simulink model "two_parallel_half_model_simscape"  (R2023b)
settings: Solver=ode1be  StartTime=0.0  StopTime=simlength  FixedStep=ts_sim  MaxStep=ts_sim
values from neighbouring files (symbols this model uses):
  fPWM_INV = 10e3    (= 10000)    [init_model.m]
  I_FS = Iout_ac_rms_nom * sqrt(2) * margin_factor    [init_model.m]
  ki_i_inv = 18    [init_model.m]
  ki_v_inv = 12.5    [init_model.m]
  kp_i_inv = 0.1    [init_model.m]
  kp_v_inv = 0.1    [init_model.m]
  LFu_ac = 125e-6*2    (= 0.00025)    [init_model.m]
  omega_grid = frequency_grid*2*pi    (= 314.159265359)    [init_model.m]
  RLFu_ac = 2e-3    (= 0.002)    [init_model.m]
  tc = ts_inv/200    (= 5e-07)    [init_model.m]
  ts_afe = ts_inv    (= 0.0001)    [init_model.m]
  ts_inv = tPWM_INV    (= 0.0001)    [init_model.m]
  ts_zvs = tPWM_ZVS*2    (= 0.0001)    [init_model.m]
  V_FS = Vout_dc_nom * margin_factor    (= 943)    [init_model.m]
  Vout_dc_nom = 820    [init_model.m]
undefined symbols (not defined in the file or in its folder): magnitude
libraries: fl_lib x43, nesl_utility x17
(part 2 of 2)

== system two_parallel_half_model_simscape/inverter_modB/single phase inverter/switch_1 ==
  Diode : fl_lib/Electrical/Electrical Elements/Diode  Vf=Vdon_diode V  Ron=Rdon_diode Ohm  Goff=1e-8 1/Ohm  i_specify=off  i_priority=None  i=0 A  i_nominal_specify=off  i_nominal_unit=A  i_nominal_value=1  v_specify=off  v_priority=None  v=0 V  v_nominal_specify=off  v_nominal_unit=V  v_nominal_value=1
  Switch : fl_lib/Electrical/Electrical Elements/Switch  R_closed=Ron Ohm  G_open=1e-8 1/Ohm  Threshold=7.5  i_specify=off  i_priority=None  i=0 A  i_nominal_specify=off  i_nominal_unit=A  i_nominal_value=1  v_specify=off  v_priority=None  v=0 V  v_nominal_specify=off  v_nominal_unit=V  v_nominal_value=1
  G : PMIOPort  Side=Left
  C : PMIOPort  Port=2  Side=Left
  E : PMIOPort  Port=3  Side=Right
  connections:
  Diode/LConn1 -- E/RConn1 -- Switch/LConn1
  Switch/RConn1 -- G/RConn1
  Diode/RConn1 -- C/RConn1 -- Switch/RConn2

== system two_parallel_half_model_simscape/inverter_modB/single phase inverter/switch_2 ==
  Diode : fl_lib/Electrical/Electrical Elements/Diode  Vf=Vdon_diode V  Ron=Rdon_diode Ohm  Goff=1e-8 1/Ohm  i_specify=off  i_priority=None  i=0 A  i_nominal_specify=off  i_nominal_unit=A  i_nominal_value=1  v_specify=off  v_priority=None  v=0 V  v_nominal_specify=off  v_nominal_unit=V  v_nominal_value=1
  Switch : fl_lib/Electrical/Electrical Elements/Switch  R_closed=Ron Ohm  G_open=1e-8 1/Ohm  Threshold=7.5  i_specify=off  i_priority=None  i=0 A  i_nominal_specify=off  i_nominal_unit=A  i_nominal_value=1  v_specify=off  v_priority=None  v=0 V  v_nominal_specify=off  v_nominal_unit=V  v_nominal_value=1
  G : PMIOPort  Side=Left
  C : PMIOPort  Port=2  Side=Left
  E : PMIOPort  Port=3  Side=Right
  connections:
  Switch/RConn2 -- C/RConn1 -- Diode/RConn1
  Switch/RConn1 -- G/RConn1
  Switch/LConn1 -- E/RConn1 -- Diode/LConn1

== system two_parallel_half_model_simscape/inverter_modB/single phase inverter/switch_3 ==
  Diode : fl_lib/Electrical/Electrical Elements/Diode  Vf=Vdon_diode V  Ron=Rdon_diode Ohm  Goff=1e-8 1/Ohm  i_specify=off  i_priority=None  i=0 A  i_nominal_specify=off  i_nominal_unit=A  i_nominal_value=1  v_specify=off  v_priority=None  v=0 V  v_nominal_specify=off  v_nominal_unit=V  v_nominal_value=1
  Switch : fl_lib/Electrical/Electrical Elements/Switch  R_closed=Ron Ohm  G_open=1e-8 1/Ohm  Threshold=7.5  i_specify=off  i_priority=None  i=0 A  i_nominal_specify=off  i_nominal_unit=A  i_nominal_value=1  v_specify=off  v_priority=None  v=0 V  v_nominal_specify=off  v_nominal_unit=V  v_nominal_value=1
  G : PMIOPort  Side=Left
  C : PMIOPort  Port=2  Side=Left
  E : PMIOPort  Port=3  Side=Right
  connections:
  Diode/LConn1 -- E/RConn1 -- Switch/LConn1
  Switch/RConn1 -- G/RConn1
  Diode/RConn1 -- C/RConn1 -- Switch/RConn2

== system two_parallel_half_model_simscape/inverter_modB/single phase inverter/switch_4 ==
  Diode : fl_lib/Electrical/Electrical Elements/Diode  Vf=Vdon_diode V  Ron=Rdon_diode Ohm  Goff=1e-8 1/Ohm  i_specify=off  i_priority=None  i=0 A  i_nominal_specify=off  i_nominal_unit=A  i_nominal_value=1  v_specify=off  v_priority=None  v=0 V  v_nominal_specify=off  v_nominal_unit=V  v_nominal_value=1
  Switch : fl_lib/Electrical/Electrical Elements/Switch  R_closed=Ron Ohm  G_open=1e-8 1/Ohm  Threshold=7.5  i_specify=off  i_priority=None  i=0 A  i_nominal_specify=off  i_nominal_unit=A  i_nominal_value=1  v_specify=off  v_priority=None  v=0 V  v_nominal_specify=off  v_nominal_unit=V  v_nominal_value=1
  G : PMIOPort  Side=Left
  C : PMIOPort  Port=2  Side=Left
  E : PMIOPort  Port=3  Side=Right
  connections:
  Switch/RConn2 -- C/RConn1 -- Diode/RConn1
  Switch/RConn1 -- G/RConn1
  Switch/LConn1 -- E/RConn1 -- Diode/LConn1

== system two_parallel_half_model_simscape/inverter_modB/single phase inverter control/acquisition_and_scaling_current ==
  in : Inport
  1/Ti5 : Gain  Gain=1/I_FS  SaturateOnIntegerOverflow=on  OutDataTypeStr=Inherit: Same as input  ParamDataTypeStr=Inherit: Same as input
  Unit Delay4 : UnitDelay  SampleTime=ts_inv  HasFrameUpgradeWarning=on
  Zero-Order Hold1 : ZeroOrderHold  SampleTime=ts_inv
  out : Outport
  wires:
  Unit Delay4/1 -> out/1
  Zero-Order Hold1/1 -> 1/Ti5/1
  1/Ti5/1 -> Unit Delay4/1
  in/1 -> Zero-Order Hold1/1

== system two_parallel_half_model_simscape/inverter_modB/single phase inverter control/alphabeta2dq ==
  note: va=V cos(wt)
      | vb=V cos(wt-2pi/3)
      | vc=V cos(wt+2pi/3)
  alpha : Inport
  beta : Inport  Port=2
  wt : Inport  Port=3
  Product{,1..3} (4 alike) : Product  RndMeth=Zero
  Sum : Sum
  Sum1 : Sum  Inputs=-+
  To Workspace1 : ToWorkspace  VariableName=id_pu_modB_sim  SampleTime=ts_inv
      settings: MaxDataPoints=Ns_inv
  To Workspace2 : ToWorkspace  VariableName=iq_pu_modB_sim  SampleTime=ts_inv
      settings: MaxDataPoints=Ns_inv
  Trigonometric Function : Trigonometry  Operator=cos
  Trigonometric Function1 : Trigonometry
  "d " : Outport  VectorParamsAs1DForOutWhenUnconnected=off
  "q " : Outport  Port=2  VectorParamsAs1DForOutWhenUnconnected=off
  wires:
  Sum1/1 -> "q "/1, To Workspace2/1
  [cos] -> Product3/1
  Product3/1 -> Sum1/2
  Product2/1 -> Sum1/1
  [sin] -> Product2/1
  Sum/1 -> "d "/1, To Workspace1/1
  beta/1 -> Product3/2, Product1/2
  [sin] -> Product1/1
  Product1/1 -> Sum/2
  Product/1 -> Sum/1
  alpha/1 -> Product2/2, Product/2
  [cos] -> Product/1
  Trigonometric Function1/1 -> [sin]
  Trigonometric Function/1 -> [cos]
  wt/1 -> Trigonometric Function/1, Trigonometric Function1/1

== system two_parallel_half_model_simscape/inverter_modB/single phase inverter control/dq2alphabeta ==
  d : Inport
  q : Inport  Port=2
  wt : Inport  Port=3
  Product{,1..3} (4 alike) : Product  RndMeth=Zero
  Sum : Sum  Inputs=+-
  Sum1 : Sum
  Trigonometric Function : Trigonometry  Operator=cos
  Trigonometric Function1 : Trigonometry
  alpha : Outport  VectorParamsAs1DForOutWhenUnconnected=off
  wires:
  wt/1 -> Trigonometric Function1/1, Trigonometric Function/1
  Trigonometric Function/1 -> [cos]
  Trigonometric Function1/1 -> [sin]
  [cos] -> Product/1
  d/1 -> Product/2, Product2/2
  Product/1 -> Sum/1
  Product1/1 -> Sum/2
  [sin] -> Product1/1
  q/1 -> Product1/2, Product3/2
  Sum/1 -> alpha/1
  [sin] -> Product2/1
  Product2/1 -> Sum1/1
  Product3/1 -> Sum1/2
  [cos] -> Product3/1

== system two_parallel_half_model_simscape/inverter_modB/single phase inverter control/pi_d ==
  id_tilde : Inport
  1/Ti : Gain  Gain=kp_i_inv  SaturateOnIntegerOverflow=on  OutDataTypeStr=Inherit: Same as input  ParamDataTypeStr=Inherit: Same as input
  Sum1 : Sum  Inputs=+++  SaturateOnIntegerOverflow=on
  Sum3 : Sum  Inputs=-+  SaturateOnIntegerOverflow=on
  To Workspace3 : ToWorkspace  VariableName=id_ctrl_out_modB_sim  SampleTime=ts_inv
      settings: MaxDataPoints=Ns_inv
  Unit Delay4 : UnitDelay  SampleTime=ts_inv  HasFrameUpgradeWarning=on
  kp2 : Gain  Gain=ki_i_inv*ts_inv  SaturateOnIntegerOverflow=on  OutDataTypeStr=Inherit: Same as input  ParamDataTypeStr=Inherit: Same as input
  ud_out_lim : Saturate  UpperLimit=1  LowerLimit=-1
  "ud_out_lim " : Saturate  UpperLimit=1  LowerLimit=-1
  Vd_out : Outport  VectorParamsAs1DForOutWhenUnconnected=off
  wires:
  "ud_out_lim "/1 -> Vd_out/1, To Workspace3/1
  ud_out_lim/1 -> "ud_out_lim "/1, Sum3/2
  Sum3/1 -> Unit Delay4/1
  Unit Delay4/1 -> Sum1/3
  1/Ti/1 -> Sum3/1, Sum1/1
  kp2/1 -> Sum1/2
  Sum1/1 -> ud_out_lim/1
  id_tilde/1 -> 1/Ti/1, kp2/1

== system two_parallel_half_model_simscape/inverter_modB/single phase inverter control/pi_q ==
  iq_tilde : Inport
  1/Ti : Gain  Gain=kp_i_inv  SaturateOnIntegerOverflow=on  OutDataTypeStr=Inherit: Same as input  ParamDataTypeStr=Inherit: Same as input
  Sum1 : Sum  Inputs=+++  SaturateOnIntegerOverflow=on
  Sum3 : Sum  Inputs=-+  SaturateOnIntegerOverflow=on
  To Workspace3 : ToWorkspace  VariableName=iq_ctrl_out_modB_sim  SampleTime=ts_inv
      settings: MaxDataPoints=Ns_inv
  Unit Delay4 : UnitDelay  SampleTime=ts_inv  HasFrameUpgradeWarning=on
  kp2 : Gain  Gain=ki_i_inv*ts_inv  SaturateOnIntegerOverflow=on  OutDataTypeStr=Inherit: Same as input  ParamDataTypeStr=Inherit: Same as input
  ud_out_lim : Saturate  UpperLimit=1  LowerLimit=-1
  "uq_out_lim " : Saturate  UpperLimit=1  LowerLimit=-1
  Vd_out : Outport  VectorParamsAs1DForOutWhenUnconnected=off
  wires:
  Sum1/1 -> ud_out_lim/1
  kp2/1 -> Sum1/2
  1/Ti/1 -> Sum1/1, Sum3/1
  Unit Delay4/1 -> Sum1/3
  Sum3/1 -> Unit Delay4/1
  ud_out_lim/1 -> Sum3/2, "uq_out_lim "/1
  "uq_out_lim "/1 -> To Workspace3/1, Vd_out/1
  iq_tilde/1 -> kp2/1, 1/Ti/1

== system two_parallel_half_model_simscape/inverter_modB/single phase inverter control/pwm ==
  vout : Inport
  Constant : Constant  Value=pi/12
  Constant1 : Constant
  Constant2 : Constant
  Constant3 : Constant
  Gain1 : Gain  Gain=1/2
  Gain2 : Gain
  Gain3 : Gain  Gain=1/2
  Gain4 : Gain  Gain=-1
  PWM generator 1 : Subsystem  mask{f=fPWM_INV, m_up=1, m_low=0, dead_time=0, pos_cmd_gate=15, neg_cmd_gate=-10, polarity=-1}
      mask prompts: f "Frequency (Hz)"; m_up "Max Input Modulation Value"; m_low "Min Input Modulation Value"; dead_time "Dead Time (s)"; pos_cmd_gate "Positive Gate Voltage (V)"; neg_cmd_gate "Negative Gate Voltage (V)"; polarity "Polarity (pu)"
  PWM generator 2 : Subsystem  mask{f=fPWM_INV, m_up=1, m_low=0, dead_time=0, pos_cmd_gate=15, neg_cmd_gate=-10, polarity=-1}
      mask prompts: f "Frequency (Hz)"; m_up "Max Input Modulation Value"; m_low "Min Input Modulation Value"; dead_time "Dead Time (s)"; pos_cmd_gate "Positive Gate Voltage (V)"; neg_cmd_gate "Negative Gate Voltage (V)"; polarity "Polarity (pu)"
  Sum : Sum  Inputs=|++
  Sum1 : Sum  Inputs=|++
  m1_top : Outport
  m1_bottom : Outport  Port=2
  m2_top : Outport  Port=3
  m2_bottom : Outport  Port=4
  wires:
  PWM generator 1/1(m1) -> m1_top/1  "gate_cmd_Q1"
  PWM generator 1/2(m2) -> m1_bottom/1  "gate_cmd_Q2"
  PWM generator 2/2(m2) -> m2_bottom/1  "gate_cmd_Q2"
  PWM generator 2/1(m1) -> m2_top/1  "gate_cmd_Q1"
  Constant/1 -> PWM generator 2/2(phase), PWM generator 1/2(phase)
  Constant1/1 -> PWM generator 2/3(polarity_input), PWM generator 1/3(polarity_input)
  Gain2/1 -> Sum/1
  Sum/1 -> Gain1/1
  Constant2/1 -> Sum/2
  Gain1/1 -> PWM generator 1/1(m_index)
  Constant3/1 -> Sum1/2
  Sum1/1 -> Gain3/1
  Gain4/1 -> Sum1/1
  Gain3/1 -> PWM generator 2/1(m_index)
  vout/1 -> Gain4/1, Gain2/1

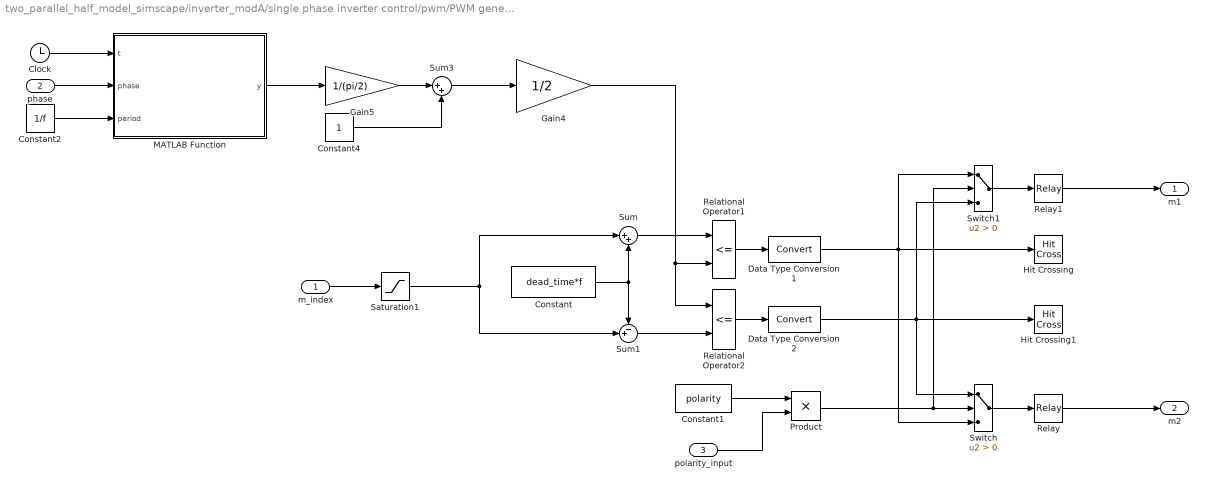
== system two_parallel_half_model_simscape/inverter_modA/single phase inverter control/pwm/PWM generator 1 ==
  m_index : Inport
  phase : Inport  Port=2
  polarity_input : Inport  Port=3
  Clock : Clock
  Constant : Constant  Value=dead_time*f
  Constant1 : Constant  Value=polarity
  Constant2 : Constant  Value=1/f
  Constant4 : Constant
  Data Type Conversion1 : DataTypeConversion
  Data Type Conversion2 : DataTypeConversion
  Gain4 : Gain  Gain=1/2
  Gain5 : Gain  Gain=1/(pi/2)
  Hit Crossing : HitCross  ShowOutputPort=off
  Hit Crossing1 : HitCross  ShowOutputPort=off
  MATLAB Function : MATLAB Function  TreatAsAtomicUnit=on
  Product : Product
  Relational Operator1 : RelationalOperator  Operator=<=  InputSameDT=off
  Relational Operator2 : RelationalOperator  Operator=<=  InputSameDT=off
  Relay : Relay  OnOutputValue=pos_cmd_gate  OffOutputValue=neg_cmd_gate
  Relay1 : Relay  OnOutputValue=pos_cmd_gate  OffOutputValue=neg_cmd_gate
  Saturation1 : Saturate  UpperLimit=m_up  LowerLimit=m_low
  Sum : Sum  Inputs=|++  SaturateOnIntegerOverflow=on
  Sum1 : Sum  Inputs=-+|  SaturateOnIntegerOverflow=on
  Sum3 : Sum  Inputs=|++
  Switch : Switch  Criteria=u2 > Threshold  SaturateOnIntegerOverflow=off  InputSameDT=off
  Switch1 : Switch  Criteria=u2 > Threshold  SaturateOnIntegerOverflow=off  InputSameDT=off
  m1 : Outport
  m2 : Outport  Port=2
  wires:
  Relational Operator1/1 -> Data Type Conversion1/1
  m_index/1 -> Saturation1/1
  Relational Operator2/1 -> Data Type Conversion2/1
  Data Type Conversion2/1 -> Switch/1, Switch1/3, Hit Crossing1/1
  Constant/1 -> Sum/2, Sum1/1
  Saturation1/1 -> Sum/1, Sum1/2
  Sum/1 -> Relational Operator1/1
  Sum1/1 -> Relational Operator2/2
  Gain4/1 -> Relational Operator2/1, Relational Operator1/2
  Data Type Conversion1/1 -> Hit Crossing/1, Switch/3, Switch1/1
  Switch/1 -> Relay/1
  Clock/1 -> MATLAB Function/1(t)
  Constant2/1 -> MATLAB Function/3(period)
  phase/1 -> MATLAB Function/2(phase)
  MATLAB Function/1(y) -> Gain5/1
  Gain5/1 -> Sum3/1
  Sum3/1 -> Gain4/1
  Constant4/1 -> Sum3/2
  Relay/1 -> m2/1
  Product/1 -> Switch1/2, Switch/2
  Switch1/1 -> Relay1/1
  Relay1/1 -> m1/1
  Constant1/1 -> Product/1
  polarity_input/1 -> Product/2

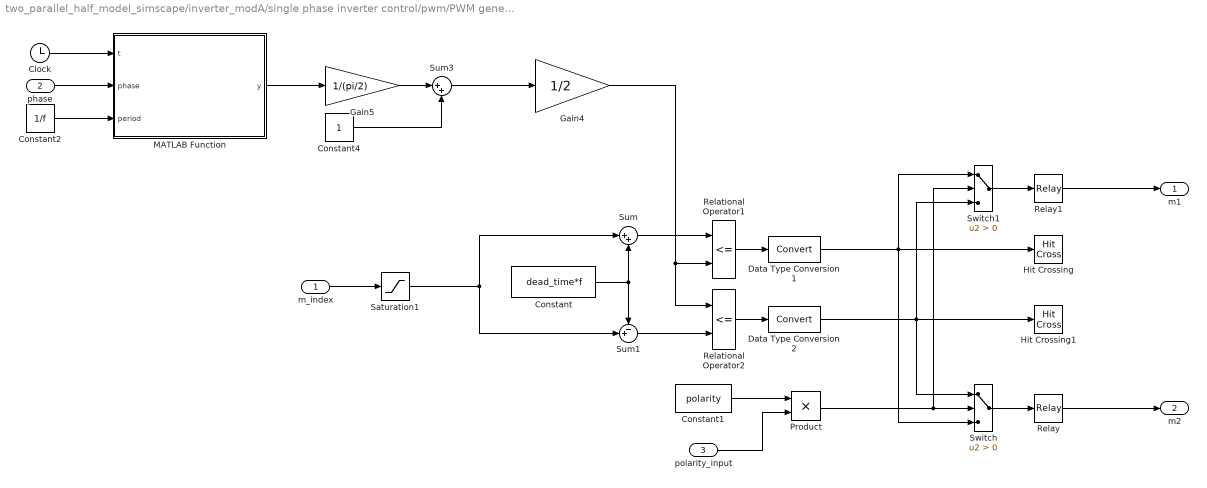
== system two_parallel_half_model_simscape/inverter_modA/single phase inverter control/pwm/PWM generator 2 ==
  m_index : Inport
  phase : Inport  Port=2
  polarity_input : Inport  Port=3
  Clock : Clock
  Constant : Constant  Value=dead_time*f
  Constant1 : Constant  Value=polarity
  Constant2 : Constant  Value=1/f
  Constant4 : Constant
  Data Type Conversion1 : DataTypeConversion
  Data Type Conversion2 : DataTypeConversion
  Gain4 : Gain  Gain=1/2
  Gain5 : Gain  Gain=1/(pi/2)
  Hit Crossing : HitCross  ShowOutputPort=off
  Hit Crossing1 : HitCross  ShowOutputPort=off
  MATLAB Function : MATLAB Function  TreatAsAtomicUnit=on
  Product : Product
  Relational Operator1 : RelationalOperator  Operator=<=  InputSameDT=off
  Relational Operator2 : RelationalOperator  Operator=<=  InputSameDT=off
  Relay : Relay  OnOutputValue=pos_cmd_gate  OffOutputValue=neg_cmd_gate
  Relay1 : Relay  OnOutputValue=pos_cmd_gate  OffOutputValue=neg_cmd_gate
  Saturation1 : Saturate  UpperLimit=m_up  LowerLimit=m_low
  Sum : Sum  Inputs=|++  SaturateOnIntegerOverflow=on
  Sum1 : Sum  Inputs=-+|  SaturateOnIntegerOverflow=on
  Sum3 : Sum  Inputs=|++
  Switch : Switch  Criteria=u2 > Threshold  SaturateOnIntegerOverflow=off  InputSameDT=off
  Switch1 : Switch  Criteria=u2 > Threshold  SaturateOnIntegerOverflow=off  InputSameDT=off
  m1 : Outport
  m2 : Outport  Port=2
  wires:
  polarity_input/1 -> Product/2
  Constant1/1 -> Product/1
  Relay1/1 -> m1/1
  Switch1/1 -> Relay1/1
  Product/1 -> Switch/2, Switch1/2
  Relay/1 -> m2/1
  Constant4/1 -> Sum3/2
  Sum3/1 -> Gain4/1
  Gain5/1 -> Sum3/1
  MATLAB Function/1(y) -> Gain5/1
  phase/1 -> MATLAB Function/2(phase)
  Constant2/1 -> MATLAB Function/3(period)
  Clock/1 -> MATLAB Function/1(t)
  Switch/1 -> Relay/1
  Data Type Conversion1/1 -> Switch1/1, Switch/3, Hit Crossing/1
  Gain4/1 -> Relational Operator1/2, Relational Operator2/1
  Sum1/1 -> Relational Operator2/2
  Sum/1 -> Relational Operator1/1
  Saturation1/1 -> Sum1/2, Sum/1
  Constant/1 -> Sum1/1, Sum/2
  Data Type Conversion2/1 -> Hit Crossing1/1, Switch1/3, Switch/1
  Relational Operator2/1 -> Data Type Conversion2/1
  m_index/1 -> Saturation1/1
  Relational Operator1/1 -> Data Type Conversion1/1

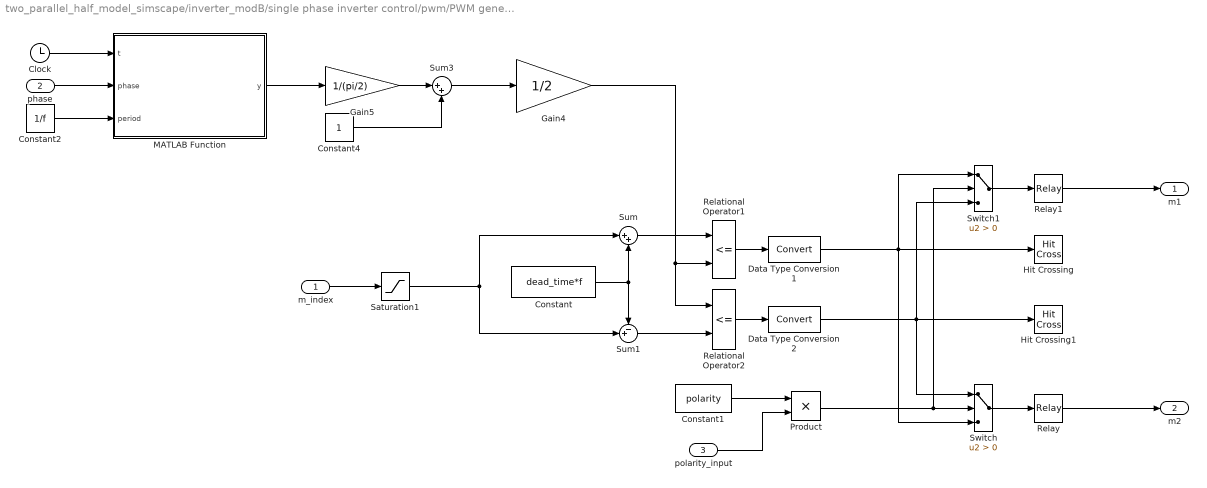
== system two_parallel_half_model_simscape/inverter_modB/single phase inverter control/pwm/PWM generator 1 ==
  m_index : Inport
  phase : Inport  Port=2
  polarity_input : Inport  Port=3
  Clock : Clock
  Constant : Constant  Value=dead_time*f
  Constant1 : Constant  Value=polarity
  Constant2 : Constant  Value=1/f
  Constant4 : Constant
  Data Type Conversion1 : DataTypeConversion
  Data Type Conversion2 : DataTypeConversion
  Gain4 : Gain  Gain=1/2
  Gain5 : Gain  Gain=1/(pi/2)
  Hit Crossing : HitCross  ShowOutputPort=off
  Hit Crossing1 : HitCross  ShowOutputPort=off
  MATLAB Function : MATLAB Function  TreatAsAtomicUnit=on
  Product : Product
  Relational Operator1 : RelationalOperator  Operator=<=  InputSameDT=off
  Relational Operator2 : RelationalOperator  Operator=<=  InputSameDT=off
  Relay : Relay  OnOutputValue=pos_cmd_gate  OffOutputValue=neg_cmd_gate
  Relay1 : Relay  OnOutputValue=pos_cmd_gate  OffOutputValue=neg_cmd_gate
  Saturation1 : Saturate  UpperLimit=m_up  LowerLimit=m_low
  Sum : Sum  Inputs=|++  SaturateOnIntegerOverflow=on
  Sum1 : Sum  Inputs=-+|  SaturateOnIntegerOverflow=on
  Sum3 : Sum  Inputs=|++
  Switch : Switch  Criteria=u2 > Threshold  SaturateOnIntegerOverflow=off  InputSameDT=off
  Switch1 : Switch  Criteria=u2 > Threshold  SaturateOnIntegerOverflow=off  InputSameDT=off
  m1 : Outport
  m2 : Outport  Port=2
  wires:
  Relational Operator1/1 -> Data Type Conversion1/1
  m_index/1 -> Saturation1/1
  Relational Operator2/1 -> Data Type Conversion2/1
  Data Type Conversion2/1 -> Switch/1, Switch1/3, Hit Crossing1/1
  Constant/1 -> Sum/2, Sum1/1
  Saturation1/1 -> Sum/1, Sum1/2
  Sum/1 -> Relational Operator1/1
  Sum1/1 -> Relational Operator2/2
  Gain4/1 -> Relational Operator2/1, Relational Operator1/2
  Data Type Conversion1/1 -> Hit Crossing/1, Switch/3, Switch1/1
  Switch/1 -> Relay/1
  Clock/1 -> MATLAB Function/1(t)
  Constant2/1 -> MATLAB Function/3(period)
  phase/1 -> MATLAB Function/2(phase)
  MATLAB Function/1(y) -> Gain5/1
  Gain5/1 -> Sum3/1
  Sum3/1 -> Gain4/1
  Constant4/1 -> Sum3/2
  Relay/1 -> m2/1
  Product/1 -> Switch1/2, Switch/2
  Switch1/1 -> Relay1/1
  Relay1/1 -> m1/1
  Constant1/1 -> Product/1
  polarity_input/1 -> Product/2

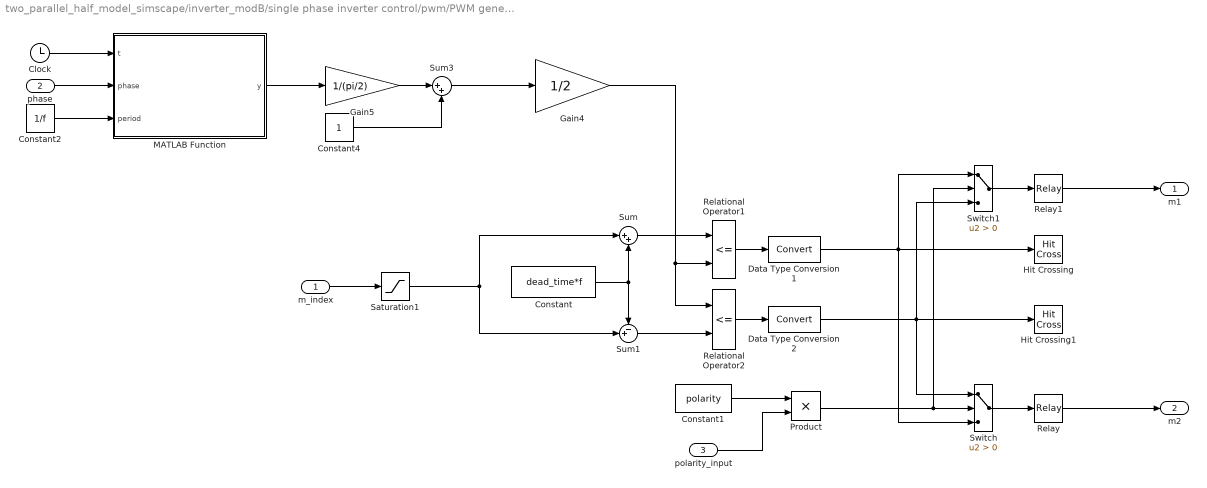
== system two_parallel_half_model_simscape/inverter_modB/single phase inverter control/pwm/PWM generator 2 ==
  m_index : Inport
  phase : Inport  Port=2
  polarity_input : Inport  Port=3
  Clock : Clock
  Constant : Constant  Value=dead_time*f
  Constant1 : Constant  Value=polarity
  Constant2 : Constant  Value=1/f
  Constant4 : Constant
  Data Type Conversion1 : DataTypeConversion
  Data Type Conversion2 : DataTypeConversion
  Gain4 : Gain  Gain=1/2
  Gain5 : Gain  Gain=1/(pi/2)
  Hit Crossing : HitCross  ShowOutputPort=off
  Hit Crossing1 : HitCross  ShowOutputPort=off
  MATLAB Function : MATLAB Function  TreatAsAtomicUnit=on
  Product : Product
  Relational Operator1 : RelationalOperator  Operator=<=  InputSameDT=off
  Relational Operator2 : RelationalOperator  Operator=<=  InputSameDT=off
  Relay : Relay  OnOutputValue=pos_cmd_gate  OffOutputValue=neg_cmd_gate
  Relay1 : Relay  OnOutputValue=pos_cmd_gate  OffOutputValue=neg_cmd_gate
  Saturation1 : Saturate  UpperLimit=m_up  LowerLimit=m_low
  Sum : Sum  Inputs=|++  SaturateOnIntegerOverflow=on
  Sum1 : Sum  Inputs=-+|  SaturateOnIntegerOverflow=on
  Sum3 : Sum  Inputs=|++
  Switch : Switch  Criteria=u2 > Threshold  SaturateOnIntegerOverflow=off  InputSameDT=off
  Switch1 : Switch  Criteria=u2 > Threshold  SaturateOnIntegerOverflow=off  InputSameDT=off
  m1 : Outport
  m2 : Outport  Port=2
  wires:
  polarity_input/1 -> Product/2
  Constant1/1 -> Product/1
  Relay1/1 -> m1/1
  Switch1/1 -> Relay1/1
  Product/1 -> Switch/2, Switch1/2
  Relay/1 -> m2/1
  Constant4/1 -> Sum3/2
  Sum3/1 -> Gain4/1
  Gain5/1 -> Sum3/1
  MATLAB Function/1(y) -> Gain5/1
  phase/1 -> MATLAB Function/2(phase)
  Constant2/1 -> MATLAB Function/3(period)
  Clock/1 -> MATLAB Function/1(t)
  Switch/1 -> Relay/1
  Data Type Conversion1/1 -> Switch1/1, Switch/3, Hit Crossing/1
  Gain4/1 -> Relational Operator1/2, Relational Operator2/1
  Sum1/1 -> Relational Operator2/2
  Sum/1 -> Relational Operator1/1
  Saturation1/1 -> Sum1/2, Sum/1
  Constant/1 -> Sum1/1, Sum/2
  Data Type Conversion2/1 -> Hit Crossing1/1, Switch1/3, Switch/1
  Relational Operator2/1 -> Data Type Conversion2/1
  m_index/1 -> Saturation1/1
  Relational Operator1/1 -> Data Type Conversion1/1

== matlab function two_parallel_half_model_simscape/inverter_modA/single phase inverter control/pwm/PWM generator 2/MATLAB Function ==
  data: t input; y output; phase input; period input
function y = trgo(t,phase,period)
x = sin(2*pi/period*t - phase - pi/2);
y = asin(x);

== matlab function two_parallel_half_model_simscape/inverter_modB/single phase inverter control/flt_dq_d_i1 ==
  data: input input; y output
function y  = flt_dq_d(input)

FLTD2Q_B1 = 0.000966531084866133;
FLTD2Q_B2 = 0.000946498544476605;
FLTD2Q_A1 = -1.93814485260962;
FLTD2Q_A2 = 0.939101367424292;

    persistent x1 x2 y1 y2

    if isempty(x1)
        x1=0;
        x2=0;
        y1=0;
        y2=0;
    end


    o = x1 * FLTD2Q_B1 + x2 * FLTD2Q_B2 - y1 * FLTD2Q_A1 - y2 * FLTD2Q_A2;
    x2 = x1;
    x1 = input;
    y2 = y1;
    y1 = o;
	y = o;
end

== matlab function two_parallel_half_model_simscape/inverter_modA/phase_gen/bounder1 ==
  data: u input; y output
function y = bounder(u)
    
    y = -pi + mod(u+3*pi,2*pi);
end

== matlab function two_parallel_half_model_simscape/inverter_modA/single phase inverter control/flt_dq_d_i ==
  data: input input; y output
function y  = flt_dq_d(input)

FLTD2Q_B1 = 0.000966531084866133;
FLTD2Q_B2 = 0.000946498544476605;
FLTD2Q_A1 = -1.93814485260962;
FLTD2Q_A2 = 0.939101367424292;

    persistent x1 x2 y1 y2

    if isempty(x1)
        x1=0;
        x2=0;
        y1=0;
        y2=0;
    end


    o = x1 * FLTD2Q_B1 + x2 * FLTD2Q_B2 - y1 * FLTD2Q_A1 - y2 * FLTD2Q_A2;
    x2 = x1;
    x1 = input;
    y2 = y1;
    y1 = o;
	y = o;
end

== matlab function two_parallel_half_model_simscape/inverter_modA/single phase inverter control/flt_dq_d_u ==
  data: input input; y output
function y  = flt_dq_d(input)

FLTD2Q_B1 = 0.000966531084866133;
FLTD2Q_B2 = 0.000946498544476605;
FLTD2Q_A1 = -1.93814485260962;
FLTD2Q_A2 = 0.939101367424292;

    persistent x1 x2 y1 y2

    if isempty(x1)
        x1=0;
        x2=0;
        y1=0;
        y2=0;
    end


    o = x1 * FLTD2Q_B1 + x2 * FLTD2Q_B2 - y1 * FLTD2Q_A1 - y2 * FLTD2Q_A2;
    x2 = x1;
    x1 = input;
    y2 = y1;
    y1 = o;
	y = o;
end

== matlab function two_parallel_half_model_simscape/inverter_modB/single phase inverter control/flt_dq_d_i ==
  data: input input; y output
function y  = flt_dq_d(input)

FLTD2Q_B1 = 0.000966531084866133;
FLTD2Q_B2 = 0.000946498544476605;
FLTD2Q_A1 = -1.93814485260962;
FLTD2Q_A2 = 0.939101367424292;

    persistent x1 x2 y1 y2

    if isempty(x1)
        x1=0;
        x2=0;
        y1=0;
        y2=0;
    end


    o = x1 * FLTD2Q_B1 + x2 * FLTD2Q_B2 - y1 * FLTD2Q_A1 - y2 * FLTD2Q_A2;
    x2 = x1;
    x1 = input;
    y2 = y1;
    y1 = o;
	y = o;
end

== matlab function two_parallel_half_model_simscape/inverter_modB/phase_gen/bounder1 ==
  data: u input; y output
function y = bounder(u)
    
    y = -pi + mod(u+3*pi,2*pi);
end

== matlab function two_parallel_half_model_simscape/inverter_modB/single phase inverter control/pwm/PWM generator 1/MATLAB Function ==
  data: t input; y output; phase input; period input
function y = trgo(t,phase,period)
x = sin(2*pi/period*t - phase - pi/2);
y = asin(x);

== matlab function two_parallel_half_model_simscape/inverter_modB/single phase inverter control/pwm/PWM generator 2/MATLAB Function ==
  data: t input; y output; phase input; period input
function y = trgo(t,phase,period)
x = sin(2*pi/period*t - phase - pi/2);
y = asin(x);

== matlab function two_parallel_half_model_simscape/inverter_modA/single phase inverter control/pwm/PWM generator 1/MATLAB Function ==
  data: t input; y output; phase input; period input
function y = trgo(t,phase,period)
x = sin(2*pi/period*t - phase - pi/2);
y = asin(x);
